simulink model "P_2_1_e_Kompeticio_modell"  (R2021b)
settings: Solver=VariableStepAuto  StartTime=0.0  StopTime=50  RelTol=1e-3
settings Model: Creator=davidpaksi  LastModifiedBy=davidpaksi

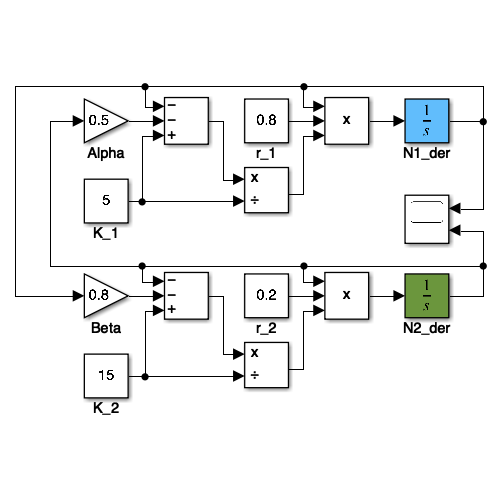
[thumbnail: Simulink's stored preview of the top-level diagram]
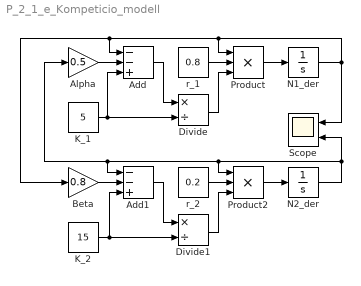
== system P_2_1_e_Kompeticio_modell ==
  Add : Sum  Inputs=--+
  Add1 : Sum  Inputs=--+
  Alpha : Gain  Gain=0.5
  Beta : Gain  Gain=0.8
  Divide : Product  Inputs=*/
  Divide1 : Product  Inputs=*/
  K_1 : Constant  Value=5
  K_2 : Constant  Value=15
  N1_der : Integrator  InitialCondition=2
  N2_der : Integrator  InitialCondition=0.5
  Product : Product  Inputs=3
  Product2 : Product  Inputs=3
  Scope : Scope  NumInputPorts=2
  r_1 : Constant  Value=0.8
  r_2 : Constant  Value=0.2
  wires:
  Product/1 -> N1_der/1
  r_1/1 -> Product/2
  N1_der/1 -> Scope/1, Beta/1, Add/1, Product/1
  Divide/1 -> Product/3
  Add/1 -> Divide/1
  N2_der/1 -> Scope/2, Alpha/1, Add1/1, Product2/1
  Product2/1 -> N2_der/1
  Divide1/1 -> Product2/3
  K_2/1 -> Divide1/2, Add1/3
  Add1/1 -> Divide1/1
  Alpha/1 -> Add/2
  K_1/1 -> Add/3, Divide/2
  r_2/1 -> Product2/2
  Beta/1 -> Add1/2
